simulink model "FLCU_Gauging_Test_Harness_Temperature"  (R2019b)
settings: Solver=FixedStepAuto  StartTime=0.0  StopTime=10  FixedStep=0.02  RelTol=1e-3
settings Model: DataDictionary=FLCU_Gauging.sldd  Creator=aymanouchker  LastModifiedBy=aymanouchker
settings DataIOCC: SignalLoggingName=BusData
settings OptimizationCC: DefaultParameterBehavior=Inlined  UseDivisionForNetSlopeComputation=on  GainParamInheritBuiltInType=on  UseFloatMulNetSlope=on  DefaultUnderspecifiedDataType=single  UseSpecifiedMinMax=on  InlineInvariantSignals=on  EnhancedBackFolding=on  CachingGlobalReferences=on  PassReuseOutputArgsAs=Individual arguments  StateBitsets=on  DataBitsets=on  ZeroExternalMemoryAtStartup=off  ZeroInternalMemoryAtStartup=off  NoFixptDivByZeroProtection=on  EfficientFloat2IntCast=on  LifeSpan=inf  OptimizeBlockOrder=speed  DifferentSizesBufferReuse=on  EfficientTunableParamExpr=on
settings DebuggingCC: SignalInfNanChecking=warning  IntegerOverflowMsg=error  ParameterTunabilityLossMsg=error  UniqueDataStoreMsg=error  AssertControl=DisableAll  StrictBusMsg=ErrorOnBusTreatedAsVector  SFUndirectedBroadcastEventsDiag=error
settings HardwareCC: ProdBitPerInt=16  ProdBitPerPointer=16  ProdBitPerSizeT=16  ProdBitPerPtrDiffT=16  ProdLargestAtomicFloat=None  ProdWordSize=16  ProdLongLongMode=on  ProdHWDeviceType=STMicroelectronics->ST10/Super10
settings SFSimCC: CompileTimeRecursionLimit=0  EnableRuntimeRecursion=off  MATLABDynamicMemAlloc=off
settings RTWCC: SystemTargetFile=ert.tlc  TemplateMakefile=ert_default_tmf  GenerateReport=on  BuildConfiguration=Faster Runs  IncludeHyperlinkInReport=on  LaunchReport=on  GenerateTraceInfo=on  GenerateTraceReport=on  GenerateTraceReportSl=on  GenerateTraceReportSf=on  GenerateTraceReportEml=on
settings CodeAppCC: ForceParamTrailComments=on  IgnoreCustomStorageClasses=off  IgnoreTestpoints=on  OperatorAnnotations=on  SimulinkDataObjDesc=on  SFDataObjDesc=on  MATLABFcnDesc=on  InsertBlockDesc=on  StateflowObjectComments=on  MATLABSourceComments=on  EnableCustomComments=on  ReqsInCode=on
settings ERTTargetCC: TargetLangStandard=C99 (ISO)  UtilityFuncGeneration=Shared location  GenerateSampleERTMain=on  CombineSignalStateStructs=on  SuppressErrorStatus=on  SupportAbsoluteTime=off  MultiInstanceERTCode=on  CodeInterfacePackaging=Reusable function  SupportNonFinite=off  ParenthesesLevel=Maximum  CastingMode=Standards  GenerateSharedConstants=off  InlinedParameterPlacement=NonHierarchical  ERTCustomFileTemplate=example_file_process.tlc  PreserveExpressionOrder=on  PreserveIfCondition=on  EnableSignedLeftShifts=off  EnableSignedRightShifts=off

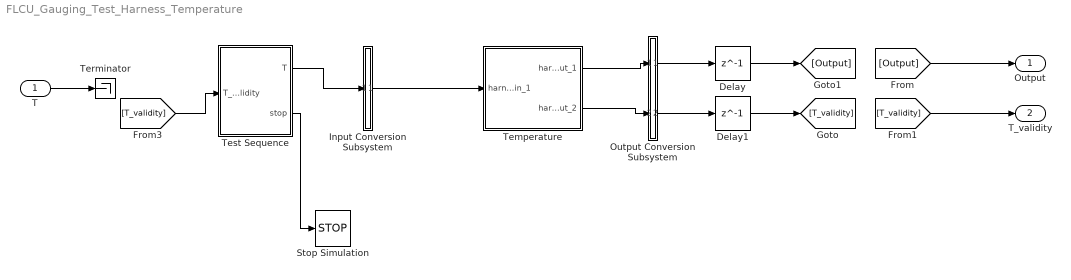
== system FLCU_Gauging_Test_Harness_Temperature ==
  T : Inport  OutDataTypeStr=double  PortDimensions=[1]  SampleTime=[-1, 0]
  Delay : Delay  DelayLength=1
  Delay1 : Delay  DelayLength=1
  Input Conversion Subsystem : Subsystem  Tag=__SLT_ICS__  Description=|
      | Signal spec.
      | and routing
      settings: AttributesFormatString=%<Description>
  Output Conversion Subsystem : Subsystem  Tag=__SLT_OCS__  Description=|
      | Signal spec.
      | and routing
      settings: AttributesFormatString=%<Description>
  Stop Simulation : Stop
  Temperature : Subsystem  Tag=__SL_testing_harness_stub_
  Terminator : Terminator
  Test Sequence : Test Sequence  TreatAsAtomicUnit=on
  Output : Outport
  T_validity : Outport  Port=2
  wires:
  Input Conversion Subsystem/1(Outport_1) -> Temperature/1(harness_in_1)
  Temperature/1(harness_out_1) -> Output Conversion Subsystem/1(Inport_1)
  Temperature/2(harness_out_2) -> Output Conversion Subsystem/2(Inport_2)
  T/1 -> Terminator/1
  Output Conversion Subsystem/1(Outport_1) -> Delay/1
  Output Conversion Subsystem/2(Outport_2) -> Delay1/1
  Delay1/1 -> [T_validity]
  Delay/1 -> [Output]
  [Output] -> Output/1
  [T_validity] -> T_validity/1
  Test Sequence/1(T) -> Input Conversion Subsystem/1(Inport_1)
  [T_validity] -> Test Sequence/1(T_validity)
  Test Sequence/2(stop) -> Stop Simulation/1

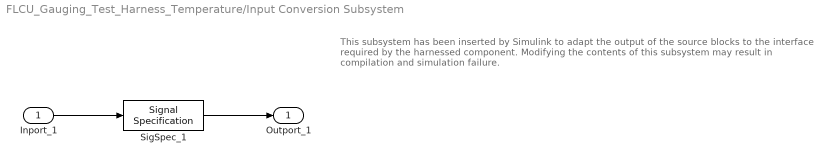
== system FLCU_Gauging_Test_Harness_Temperature/Input Conversion Subsystem ==
  note: This subsystem has been inserted by Simulink to adapt the output of the source blocks to the interface required by the harnessed component.
      |  Modifying the contents of this subsystem may result in compilation and simulation failure.
  Inport_1 : Inport
  SigSpec_1 : SignalSpecification  OutDataTypeStr=double  Unit=°C  Dimensions=[1]  SampleTime=[-1, 0]
  Outport_1 : Outport
  wires:
  SigSpec_1/1 -> Outport_1/1
  Inport_1/1 -> SigSpec_1/1

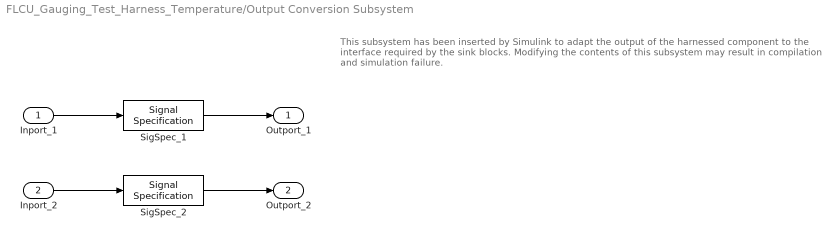
== system FLCU_Gauging_Test_Harness_Temperature/Output Conversion Subsystem ==
  note: This subsystem has been inserted by Simulink to adapt the output of the harnessed component to the interface required by the sink blocks.
      |  Modifying the contents of this subsystem may result in compilation and simulation failure.
  Inport_1 : Inport
  Inport_2 : Inport  Port=2
  SigSpec_1 : SignalSpecification  OutDataTypeStr=double  Unit=°C  Dimensions=[1]
  SigSpec_2 : SignalSpecification  OutDataTypeStr=boolean  Dimensions=[1]
  Outport_1 : Outport
  Outport_2 : Outport  Port=2
  wires:
  Inport_1/1 -> SigSpec_1/1
  SigSpec_1/1 -> Outport_1/1
  Inport_2/1 -> SigSpec_2/1
  SigSpec_2/1 -> Outport_2/1

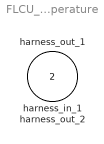
== system FLCU_Gauging_Test_Harness_Temperature/Temperature ==
  harness_in_1 : Inport
  harness_out_1 : Outport
  harness_out_2 : Outport  Port=2

== stateflow chart FLCU_Gauging_Test_Harness_Temperature/Test Sequence ==
  settings: stateMachineType=SIMPLIFIED_MACHINE
  state Initialization
    T=0;
    stop=false;
    count=0;
  state step_1
    T=1;
  state step_2
    verify(T_validity==true);
  state step_3
    T=-120;
  state step_4
    count=count+1;
    verify(T_validity==false);
  state step_5
    T=160;
  state step_6
    T=-100
  state step_7
    T=150;
  state step_8
    stop=true;
  (default) -> Initialization
  Initialization -> step_1
  step_1 -> step_2
  step_2 -> step_3
  step_3 -> step_4
  (junction 54) -> step_4
  step_4 -> (junction 39) [order 2] : [
      | count==2
      | ]
  (junction 56) -> (junction 54)
  (junction 39) -> (junction 37)
  step_4 -> (junction 44) [order 3] : [
      | count==3
      | ]
  (junction 44) -> (junction 42)
  step_4 -> (junction 49) [order 4] : [
      | count==4
      | ]
  (junction 49) -> (junction 47)
  step_4 -> step_5 [order 1] : [
      | count==1
      | ]
  step_5 -> step_4
  step_6 -> (junction 56)
  (junction 37) -> step_6
  (junction 59) -> (junction 56)
  step_7 -> (junction 59)
  (junction 42) -> step_7
  (junction 47) -> step_8
  data: T_validity input; T output; stop output; count local
